simulink model "dyn"  (R2024b)
settings: Solver=VariableStepAuto  StartTime=0.0  StopTime=10.0  RelTol=1e-3
values from neighbouring files (symbols this model uses):
  cmd = ones(6,1)* cmd_4    [MAIN.m]    (also in MAIN_exam_2025.m = ones(6,1) * cmd)
  F = [zeros(2,6);ones(1,6); row1; row2; direction * sigma]    [MAIN.m]    (also in MAIN_exam_2025.m)
  lambda = diag(ones(6,1))*0.6    [MAIN.m]    (also in MAIN_exam_2025.m = diag(ones(6,1)))
  omegab_0 = [0 0 0]'    [MAIN.m]    (also in MAIN_exam_2025.m)
  p_i_0 = [0 0 1]'    [MAIN_exam_2025.m]
  q_0 = eul2quat([0, theta_cmd, 0 ]*degToRad,'ZYX')'    [MAIN.m]    (also in MAIN_exam_2025.m = eul2quat([0, 0, 0 ]*degToRad,'XYZ')')
  UAV = include_pack(UAV,pack,1)    [MAIN.m]
  vb_0 = zeros(3,1)    [MAIN.m]    (also in MAIN_exam_2025.m = [0 0 0]')
undefined symbols (not defined in the file or in its folder): par
settings Model: Creator=ggera  LastModifiedBy=ggera

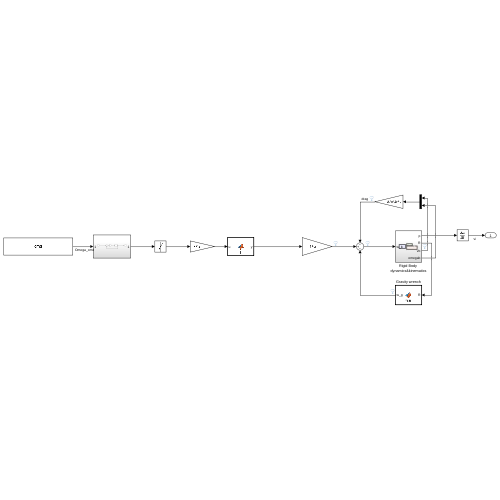
[thumbnail: Simulink's stored preview of the top-level diagram]
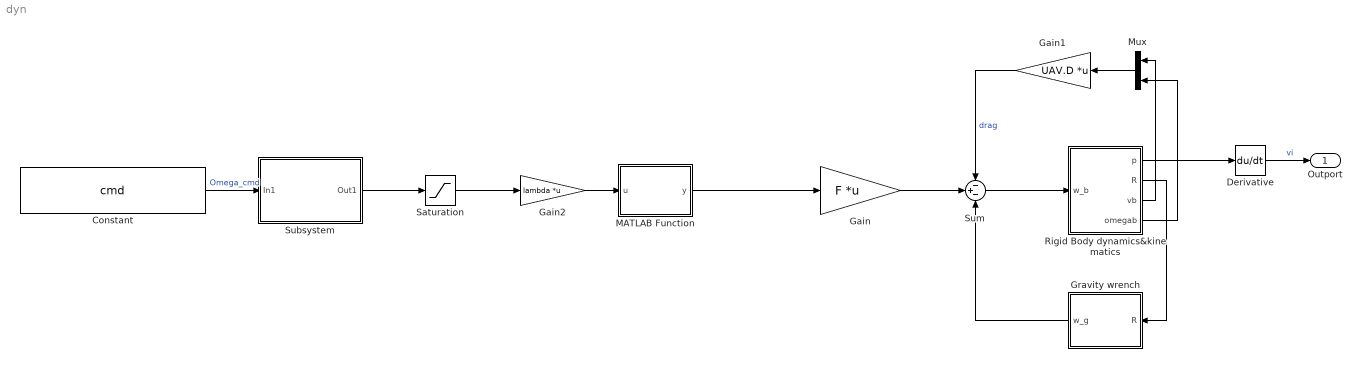
== system dyn ==
  Constant : Constant  Value=cmd
  Derivative : Derivative
  Gain : Gain  Gain=F  Multiplication=Matrix(K*u)
  Gain1 : Gain  Gain=UAV.D  Multiplication=Matrix(K*u)
  Gain2 : Gain  Gain=lambda  Multiplication=Matrix(K*u)
  Gravity wrench : MATLAB Function  TreatAsAtomicUnit=on
  MATLAB Function : MATLAB Function  TreatAsAtomicUnit=on
  Mux : Mux  Inputs=2
  "Rigid Body dynamics&kinematics " : Subsystem
  Saturation : Saturate  UpperLimit=UAV.Omega_max  LowerLimit=UAV.Omega_min
  Subsystem : Subsystem
  Sum : Sum  Inputs=-+-
  Outport : Outport
  wires:
  Gain2/1 -> MATLAB Function/1(u)
  Sum/1 -> "Rigid Body dynamics&kinematics "/1(w_b)
  Gain/1 -> Sum/2
  Gravity wrench/1(w_g) -> Sum/3
  Gain1/1 -> Sum/1  "drag"
  "Rigid Body dynamics&kinematics "/2(R) -> Gravity wrench/1(R)
  Constant/1 -> Subsystem/1(In1)  "Omega_cmd"
  Mux/1 -> Gain1/1
  MATLAB Function/1(y) -> Gain/1
  "Rigid Body dynamics&kinematics "/4(omegab) -> Mux/2
  "Rigid Body dynamics&kinematics "/3(vb) -> Mux/1
  "Rigid Body dynamics&kinematics "/1(p) -> Derivative/1
  Derivative/1 -> Outport/1  "vi"
  Subsystem/1(Out1) -> Saturation/1
  Saturation/1 -> Gain2/1

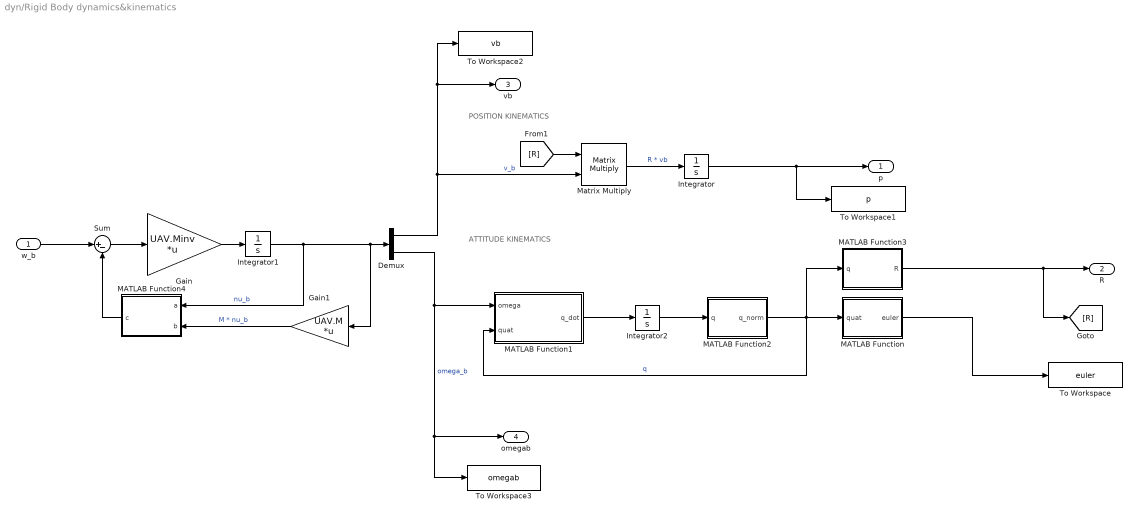
== system dyn/Rigid Body dynamics&kinematics  ==
  note: ATTITUDE KINEMATICS
  note: POSITION KINEMATICS
  w_b : Inport
  Demux : Demux  Outputs=2
  Gain : Gain  Gain=UAV.Minv  Multiplication=Matrix(K*u)
  Gain1 : Gain  Gain=UAV.M  Multiplication=Matrix(K*u)
  Integrator : Integrator  InitialCondition=p_i_0
  Integrator1 : Integrator  InitialCondition=[vb_0;omegab_0]
  Integrator2 : Integrator  InitialCondition=q_0
  MATLAB Function : MATLAB Function  TreatAsAtomicUnit=on
  MATLAB Function1 : MATLAB Function  TreatAsAtomicUnit=on
  MATLAB Function2 : MATLAB Function  TreatAsAtomicUnit=on
  MATLAB Function3 : MATLAB Function  TreatAsAtomicUnit=on
  MATLAB Function4 : MATLAB Function  TreatAsAtomicUnit=on
  Matrix Multiply : Product  Multiplication=Matrix(*)
  Sum : Sum  Inputs=|+-
  To Workspace : ToWorkspace  VariableName=euler  SaveFormat=Timeseries  SampleTime=-1
  To Workspace1 : ToWorkspace  VariableName=p  SaveFormat=Timeseries  SampleTime=-1
  To Workspace2 : ToWorkspace  VariableName=vb  SaveFormat=Timeseries  SampleTime=-1
  To Workspace3 : ToWorkspace  VariableName=omegab  SaveFormat=Timeseries  SampleTime=-1
  p : Outport
  R : Outport  Port=2
  vb : Outport  Port=3
  omegab : Outport  Port=4
  wires:
  Integrator/1 -> p/1, To Workspace1/1
  MATLAB Function1/1(q_dot) -> Integrator2/1
  MATLAB Function2/1(q_norm) -> MATLAB Function3/1(q), MATLAB Function1/2(quat), MATLAB Function/1(quat)  "q"
  MATLAB Function3/1(R) -> R/1, [R]
  Demux/1 -> vb/1, To Workspace2/1, Matrix Multiply/2  "v_b"
  Integrator1/1 -> Demux/1, Gain1/1, MATLAB Function4/1(a)  "nu_b"
  Integrator2/1 -> MATLAB Function2/1(q)
  Matrix Multiply/1 -> Integrator/1  "R * vb"
  MATLAB Function/1(euler) -> To Workspace/1
  [R] -> Matrix Multiply/1
  Gain/1 -> Integrator1/1
  Demux/2 -> omegab/1, To Workspace3/1, MATLAB Function1/1(omega)  "omega_b"
  Gain1/1 -> MATLAB Function4/2(b)  "M * nu_b"
  Sum/1 -> Gain/1
  MATLAB Function4/1(c) -> Sum/2
  w_b/1 -> Sum/1

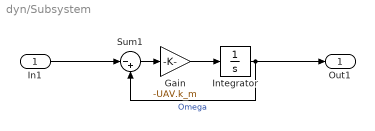
== system dyn/Subsystem ==
  In1 : Inport
  Gain : Gain  Gain=-UAV.k_m
  Integrator : Integrator  InitialCondition=cmd
  Sum1 : Sum  Inputs=|-+
  Out1 : Outport
  wires:
  Sum1/1 -> Gain/1
  Integrator/1 -> Sum1/2, Out1/1  "Omega"
  In1/1 -> Sum1/1
  Gain/1 -> Integrator/1

== matlab function dyn/Rigid Body dynamics&kinematics /MATLAB Function1 ==
  data: omega input; quat input; q_dot output
 function q_dot = quat_kin(omega, quat)
%#codegen

eta = quat(1);
eps = quat(2:4);

W=[-eps';
   skew(eps) + eta*eye(3)];

q_dot = 0.5*W*omega;

end

function S=skew(s)
S=[0  -s(3)  s(2);
    s(3)   0 -s(1);
    -s(2)  s(1)  0];
end

== matlab function dyn/Rigid Body dynamics&kinematics /MATLAB Function ==
  data: quat input; euler output
function euler = quatToEuler( quat )
%	Converts a quaternion vector to ZYX Euler angles (RPY)

euler = quat2eul(quat','ZYX');

end

== matlab function dyn/Rigid Body dynamics&kinematics /MATLAB Function2 ==
  data: q input; q_norm output
function q_norm = quat_norm( q )

norm = sqrt( q(1)^2 + q(2)^2 + q(3)^2 + q(4)^2 );

q_norm = 1/norm * q;

== matlab function dyn/Rigid Body dynamics&kinematics /MATLAB Function3 ==
  data: q input; R output
function R = fcn(q)

R = quat2rotm(q');

end

== matlab function dyn/Rigid Body dynamics&kinematics /MATLAB Function4 ==
  data: a input; c output; b input
function c = cross_six(a,b)

a_v = a(1:3);
a_omega = a(4:6);

cross_six = [crossmat(a_omega), zeros(3,3);
             crossmat(a_v), crossmat(a_omega)] ;

c = cross_six*b;

end

function S=crossmat(s)
S=[0  -s(3)  s(2);
    s(3)   0 -s(1);
    -s(2)  s(1)  0];
end

== matlab function dyn/Gravity wrench ==
  data: R input; w_g output; UAV parameter; par parameter
function w_g = fcn(R,UAV,par)

e_3 = par.e3;
g = par.g;

w_g = g*[UAV.m*R'*e_3; UAV.S*R'*e_3];

== matlab function dyn/MATLAB Function ==
  data: u input; y output; k_f parameter
function y = T(u, k_f)
    y = u;
    a = length(u);
    for i = 1:a
        y(i) = k_f * u(i)^2;
    end
end
